simulink model "sltestNormalSILEquivalenceExample"  (R2016a)
settings: Solver=ode3  StartTime=0.0  StopTime=10  FixedStep=0.01  RelTol=1e-3
Description:
  | Software-in-the-Loop Code Verification
settings Model: ExtModeAutoUpdateStatusClock=off  Creator=The MathWorks, Inc.  LastModifiedBy=The MathWorks, Inc.
settings DataIOCC: SaveFormat=Array  ReturnWorkspaceOutputs=on  SignalLoggingName=SIL_signals
settings OptimizationCC: DefaultParameterBehavior=Inlined  UseDivisionForNetSlopeComputation=on  InlineInvariantSignals=on  EnhancedBackFolding=on  BooleansAsBitfields=on  PassReuseOutputArgsAs=Individual arguments  ExpressionDepthLimit=2147483647  StateBitsets=on  DataBitsets=on  ZeroExternalMemoryAtStartup=off  ZeroInternalMemoryAtStartup=off  NoFixptDivByZeroProtection=on  EfficientFloat2IntCast=on  OptimizeModelRefInitCode=on  LifeSpan=1
settings DebuggingCC: CheckExecutionContextPreStartOutputMsg=on  CheckExecutionContextRuntimeOutputMsg=on  FcnCallInpInsideContextMsg=UseLocalSettings  AllowSymbolicDim=off  StateNameClashWarn=warning  StrictBusMsg=ErrorOnBusTreatedAsVector
settings HardwareCC: ProdBitPerPointer=32  ProdLargestAtomicInteger=Long  ProdLargestAtomicFloat=Double  ProdWordSize=32  ProdHWDeviceType=ARM Compatible->ARM Cortex  TargetBitPerLong=64  TargetBitPerPointer=64  TargetLongLongMode=on  TargetIntDivRoundTo=Zero  TargetEndianess=LittleEndian  TargetWordSize=64  TargetHWDeviceType=Generic->MATLAB Host Computer
settings ModelReferenceCC: PropagateSignalLabelsOutOfModel=off
settings RTWCC: SystemTargetFile=ert.tlc  TemplateMakefile=ert_default_tmf  GenerateReport=on  RTWVerbose=off  IncludeHyperlinkInReport=on  PortableWordSizes=on  CreateSILPILBlock=SIL  GenerateTraceInfo=on  GenerateTraceReport=on  GenerateTraceReportSl=on  GenerateTraceReportSf=on  GenerateTraceReportEml=on  GenerateCodeMetricsReport=on
settings CodeAppCC: ForceParamTrailComments=on  IgnoreCustomStorageClasses=off  IgnoreTestpoints=on  SimulinkDataObjDesc=on  CustomSymbolStrGlobalVar=rt$N$M  CustomSymbolStrType=$N$M  CustomSymbolStrFcn=$N$M$F  CustomSymbolStrMacro=$N$M  InsertBlockDesc=on  InternalIdentifier=Classic
settings ERTTargetCC: UtilityFuncGeneration=Shared location  GenerateSampleERTMain=on  IncludeMdlTerminateFcn=off  CombineSignalStateStructs=on  SupportNonFinite=off  SupportComplex=off  SupportContinuousTime=on  InlinedParameterPlacement=NonHierarchical  ERTCustomFileTemplate=example_file_process.tlc  ERTFilePackagingFormat=CompactWithDataFile  ConvertIfToSwitch=off  SuppressUnreachableDefaultCases=off
settings ConfigComp: CovModelRefEnable=Off  CovSFcnEnable=off

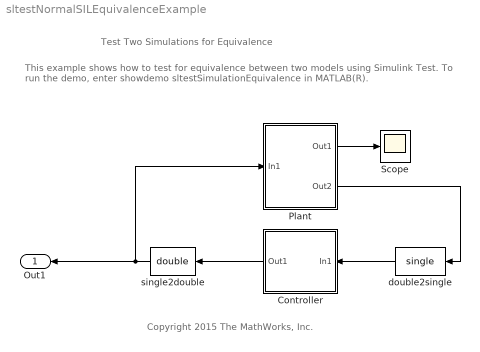
== system sltestNormalSILEquivalenceExample ==
  note: This example shows how to test for equivalence between two models using Simulink Test.
      | To run the demo, enter showdemo sltestSimulationEquivalence in MATLAB(R).
  note: Test Two Simulations for Equivalence
  note: Copyright 2015 The MathWorks, Inc.
  Controller : Subsystem  TreatAsAtomicUnit=on
      settings: RTWFcnNameOpts=Use subsystem name  RTWFileNameOpts=Use function name
  Plant : Subsystem
  Scope : Scope
  double2single : DataTypeConversion  OutDataTypeStr=single
  single2double : DataTypeConversion  OutDataTypeStr=double
  Out1 : Outport
  wires:
  Plant/1(Out1) -> Scope/1
  Plant/2(Out2) -> double2single/1
  double2single/1 -> Controller/1(In1)
  single2double/1 -> Out1/1, Plant/1(In1)
  Controller/1(Out1) -> single2double/1

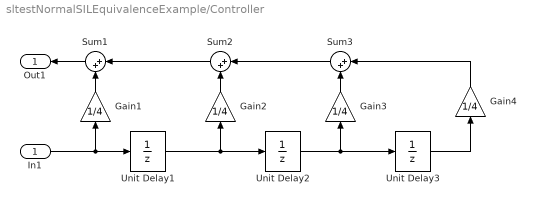
== system sltestNormalSILEquivalenceExample/Controller ==
  In1 : Inport  SampleTime=.01
  Gain{1..4} (4 alike) : Gain  Gain=1/4  SaturateOnIntegerOverflow=on  ParamDataTypeStr=Inherit: Same as input
  Sum1 : Sum  Inputs=|++  SaturateOnIntegerOverflow=on  InputSameDT=on  OutDataTypeStr=Inherit: Same as first input
  Sum2 : Sum  Inputs=|++  SaturateOnIntegerOverflow=on  InputSameDT=on  OutDataTypeStr=Inherit: Same as first input
  Sum3 : Sum  Inputs=|++  SaturateOnIntegerOverflow=on  InputSameDT=on  OutDataTypeStr=Inherit: Same as first input
  Unit Delay1 : UnitDelay  SampleTime=-1
  Unit Delay2 : UnitDelay  SampleTime=-1
  Unit Delay3 : UnitDelay  SampleTime=-1
  Out1 : Outport
  wires:
  Gain1/1 -> Sum1/2
  In1/1 -> Unit Delay1/1, Gain1/1
  Sum1/1 -> Out1/1
  Sum3/1 -> Sum2/1
  Sum2/1 -> Sum1/1
  Unit Delay1/1 -> Unit Delay2/1, Gain2/1
  Unit Delay2/1 -> Unit Delay3/1, Gain3/1
  Unit Delay3/1 -> Gain4/1
  Gain4/1 -> Sum3/1
  Gain3/1 -> Sum3/2
  Gain2/1 -> Sum2/2

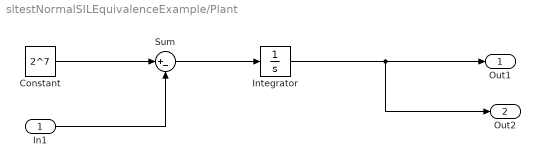
== system sltestNormalSILEquivalenceExample/Plant ==
  In1 : Inport
  Constant : Constant  Value=2^7
  Integrator : Integrator
  Sum : Sum  Inputs=|+-  SaturateOnIntegerOverflow=on  InputSameDT=on  OutDataTypeStr=Inherit: Same as first input
  Out1 : Outport
  Out2 : Outport  Port=2
  wires:
  Integrator/1 -> Out1/1, Out2/1
  Sum/1 -> Integrator/1
  Constant/1 -> Sum/1
  In1/1 -> Sum/2
